simulink model "dcmotor"  (R2021a)
settings: Solver=VariableStepAuto  StartTime=0.0  StopTime=10.0  RelTol=1e-3
undefined symbols (not defined in the file): Ion, Lithium
libraries: spsSeriesRLCBranchLib x5, spsDCMachineLib x1, spsPWMGeneratorDCDCLib x1, spsPVArrayLib x1, spsBatteryLib x1, spsCurrentMeasurementLib x1, spsDiodeLib x1, spsMosfetLib x1, spsVoltageMeasurementLib x1, spspowerguiLib x1
settings Model: Creator=Gue$t  LastModifiedBy=Gue$t

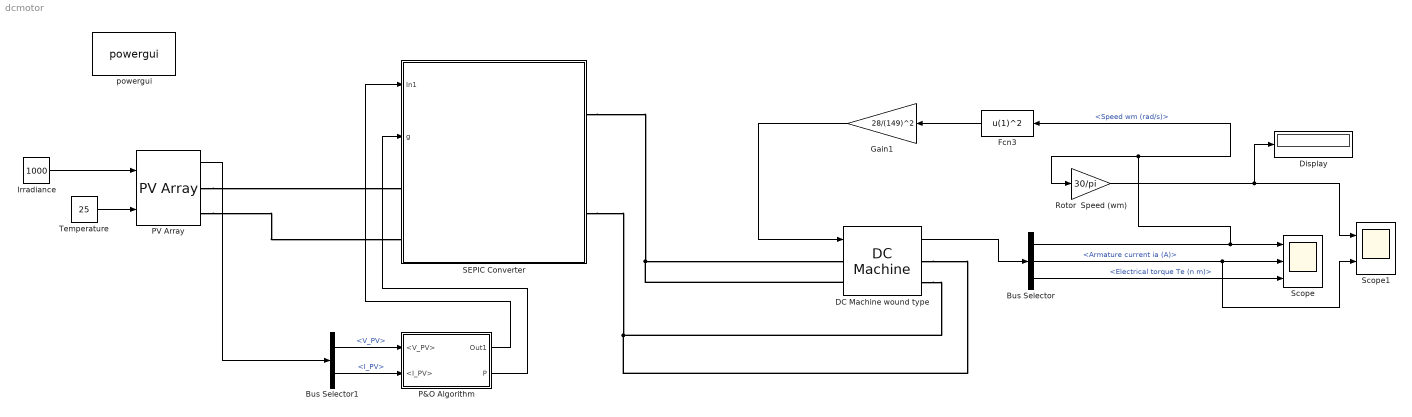
== system dcmotor ==
  Bus Selector : BusSelector  OutputSignals=Speed wm (rad/s),Armature current ia (A),Electrical torque Te (n m)
  Bus Selector1 : BusSelector  OutputSignals=V_PV,I_PV
  DC Machine wound type : spsDCMachineLib/DC Machine  PresetModel=01: 5HP 240V 1750RPM Field:300V  MechanicalLoad=Torque TL  FieldType=Wound  ShowDetailedParameters=on  MeasurementBus=off  RLa=[2.581 0.028]  RLf=[281.2 156]  Laf=0.9483  MachineConstant=Torque constant (N.m/A)  Ke=1.8  Kt=1.8  J=0.02215  Bm=0.002953  Tf=0.5161  w0=1  Ifinit=0  TsPowergui=0  TsBlock=-1
  Display : Display
  Fcn3 : Fcn  Expr=u(1)^2
  Gain1 : Gain  Gain=28/(149)^2
  Irradiance : Constant  Value=1000
  P&O Algorithm : Subsystem
  PV Array : spsPVArrayLib/PV Array  Npar=2  Nser=3  PlotType=array @ 1000 W/m2 & specified temperatures  S_vec="[ 1000  500  100 ]"  Temp_C_vec="[ 45 25  ]"  ModuleName=User-defined  PlotWhenSelected=off  Pm=224.757  Ncell=60  Voc=41.79  Isc=7.13  Vm=33.9  Im=6.63  beta_Voc_pc=-0.36099  alpha_Isc_pc=0.102  beta_Voc=-0.15086  alpha_Isc=0.0072726  IL=7.142  I0=2.6501e-10  nI=1.1299  Rsh=247.0314  Rs=0.41409  RobustModel=off  RobustCellTemperature=313.3991  BAL=on  Tc=1e-6  Tfilter=5e-5
  Rotor  Speed (wm) : Gain  Gain=30/pi
  SEPIC Converter : Subsystem
  Scope : Scope  NumInputPorts=3
  Scope1 : Scope  NumInputPorts=2
  Temperature : Constant  Value=25
  powergui : spspowerguiLib/powergui  Priority=1  SimulationMode=Discrete  SampleTime=1e-6  frequency=60  Iterations=50  frequencyindice=0  Pbase=100e6  ErrMax=1e-4  UnitsV=kV  UnitsW=MW  buscounter=0  FunctionMessages=off  echomessages=off  EnableUseOfTLC=off  CurrentSourceSwitches=off  DisableSnubberDevices=off  DisableRonSwitches=off  DisableVfSwitches=off  DisplayEquations=off  AutomaticDiscreteSolvers=off  SolverType=Tustin/Backward Euler (TBE)  Interpol=off  ExternalGateDelay=off  methode=off  Ts=100  x0status=blocks  SPID=on  SwTol=0  HookPort=off  NonlinearTolerance=0  nMaxIteration=15  ContinueOnMaxIteration=off  RestoreLinks=warning  ResistiveCurrentMeasurement=off  Frange=[0:2:500]  Ylog=off  Xlog=on  ShowGrid=off  save=off  variable=ZData  structure=0  ZoomFFT=off  StartTime=0.0  cycles=1  DisplayStyle=1  fundamental=60  FreqAxis=off  MaxFrequency=1000  frequencyindicesteady=1  RmsSteady=1  display=off
  wires:
  Bus Selector1/2 -> P&O Algorithm/2(<I_PV>)  "<I_PV>"
  PV Array/1 -> Bus Selector1/1
  Irradiance/1 -> PV Array/1
  Bus Selector1/1 -> P&O Algorithm/1(<V_PV>)  "<V_PV>"
  P&O Algorithm/2(P) -> SEPIC Converter/2(g)
  P&O Algorithm/1(Out1) -> SEPIC Converter/1(In1)
  Temperature/1 -> PV Array/2
  Bus Selector/3 -> Scope/3  "<Electrical torque Te (n m)>"
  Fcn3/1 -> Gain1/1
  Bus Selector/1 -> Fcn3/1, Rotor  Speed (wm)/1, Scope/1  "<Speed wm (rad/s)>"
  Rotor  Speed (wm)/1 -> Scope1/1, Display/1
  Bus Selector/2 -> Scope1/2, Scope/2  "<Armature current ia (A)>"
  DC Machine wound type/1 -> Bus Selector/1
  Gain1/1 -> DC Machine wound type/1
  connections:
  PV Array/RConn1 -- SEPIC Converter/LConn1
  PV Array/RConn2 -- SEPIC Converter/LConn2
  SEPIC Converter/RConn2 -- DC Machine wound type/RConn1 -- DC Machine wound type/RConn2
  SEPIC Converter/RConn1 -- DC Machine wound type/LConn2 -- DC Machine wound type/LConn1

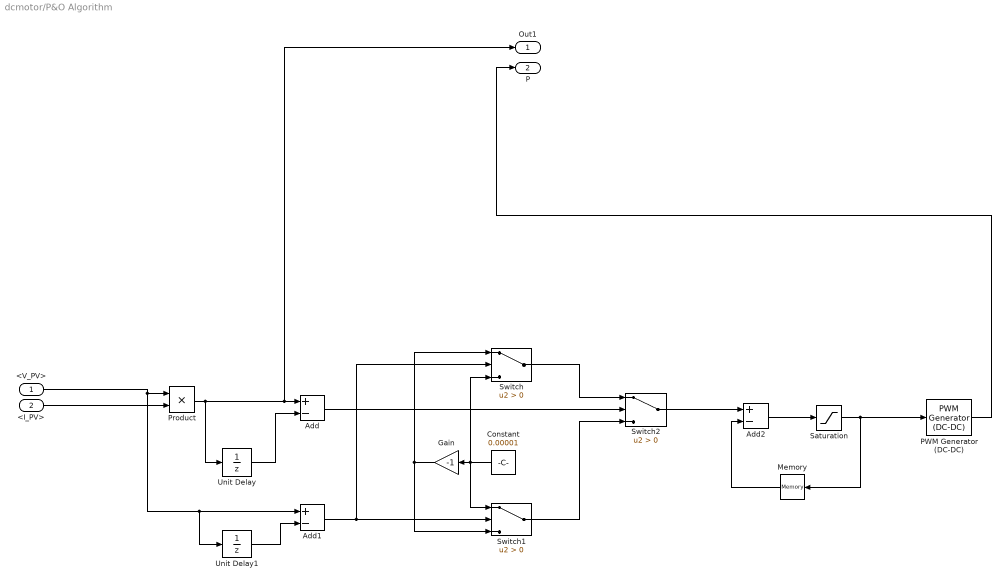
== system dcmotor/P&O Algorithm ==
  <V_PV> : Inport
  <I_PV> : Inport  Port=2
  Add : Sum  Inputs=+-
  Add1 : Sum  Inputs=+-
  Add2 : Sum  Inputs=+-
  Constant : Constant  Value=0.00001
  Gain : Gain  Gain=-1
  Memory : Memory
  PWM Generator (DC-DC) : spsPWMGeneratorDCDCLib/PWM Generator (DC-DC)  Fsw=50  Ts=0
      link override Sawtooth Generator/Model/Hit  Crossing: HitCrossingOffset=0.001
  Product : Product
  Saturation : Saturate
  Switch : Switch  Criteria=u2 > Threshold
  Switch1 : Switch  Criteria=u2 > Threshold
  Switch2 : Switch  Criteria=u2 > Threshold
  Unit Delay : UnitDelay  SampleTime=-1  HasFrameUpgradeWarning=on
  Unit Delay1 : UnitDelay  SampleTime=-1  HasFrameUpgradeWarning=on
  Out1 : Outport
  P : Outport  Port=2
  wires:
  Add1/1 -> Switch/2, Switch1/2
  Constant/1 -> Switch1/1, Switch/3, Gain/1
  Product/1 -> Out1/1, Add/1, Unit Delay/1
  Gain/1 -> Switch1/3, Switch/1
  Switch/1 -> Switch2/1
  PWM Generator (DC-DC)/1 -> P/1
  Switch2/1 -> Add2/1
  Add/1 -> Switch2/2
  Switch1/1 -> Switch2/3
  Saturation/1 -> Memory/1, PWM Generator (DC-DC)/1
  <V_PV>/1 -> Add1/1, Unit Delay1/1, Product/1
  Unit Delay1/1 -> Add1/2
  Add2/1 -> Saturation/1
  Unit Delay/1 -> Add/2
  Memory/1 -> Add2/2
  <I_PV>/1 -> Product/2

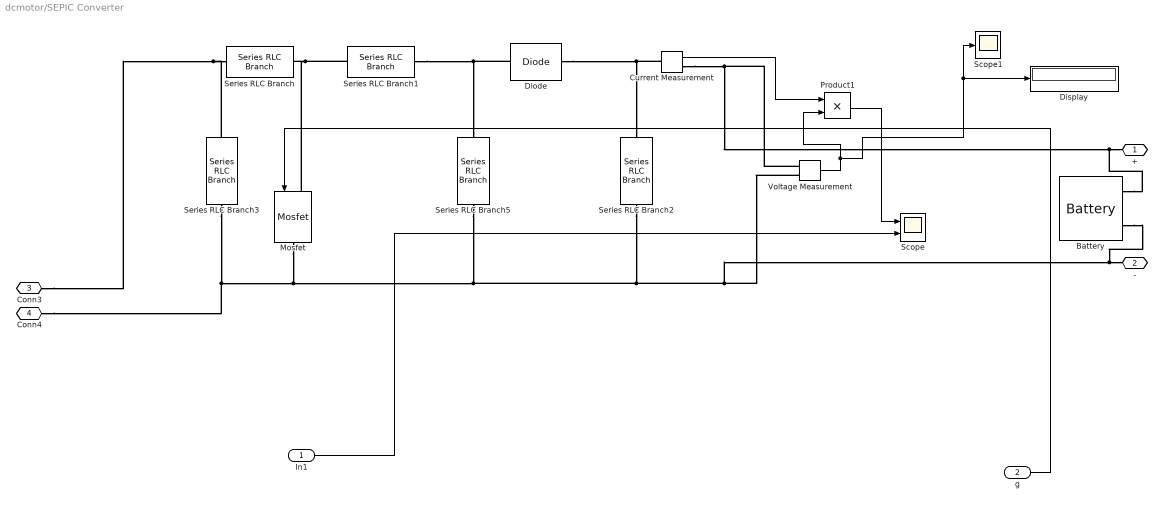
== system dcmotor/SEPIC Converter ==
  In1 : Inport
  g : Inport  Port=2
  Battery : spsBatteryLib/Battery  BatType=Lithium-Ion  ShowTempParam=off  ThermalPreset=no  ShowAgeParam=off  NomV=350  NomQ=5.4  SOC=100  Batt_Tr=30  PresetModel=on  MaxQ=5.4  MinV=262.5  FullV=407.3955  Dis_rate=2.3478  R=0.64815  Normal_OP=4.8835  expZone="[378.135     0.2653043]"  current=[6.5 13 32.5]  Units=Time  Tci=20  NomT=20  T2=-30  MaxQ2=4.8  FullV2=7.1  Normal_OP2=5.655  expZone2="[6.58           1]"  Rca=0.6  ti=2000  Dp=0  Neq0=0  Tsim=1e6  Ta1=25  Qeol=5.4*0.9  Reol=0.013333*1.2  Char_age=[2.3478, 3]  Dis_age=[2.3478, 10]  N1=1500  N2=10500  N3=1000  N4=1400  Ta2=45  N5=950
  Current Measurement : spsCurrentMeasurementLib/Current Measurement  PhasorSimulation=off  OutputType=Complex  PSBequivalent=0
  Diode : spsDiodeLib/Diode  Ron=0.001  Lon=0  Vf=0.8  IC=0  UseSnubber=0  Rs=500  Cs=250e-9  Measurements=off
  Display : Display
  Mosfet : spsMosfetLib/Mosfet  Ron=0.1  Lon=0  Rd=0.01  Vfd=0  IC=0  Rs=1e5  Cs=inf  Measurements=off
  Product1 : Product
  Scope : Scope  NumInputPorts=2
  Scope1 : Scope
  Series RLC Branch : spsSeriesRLCBranchLib/Series RLC Branch  LConnTagsString=__new0  RConnTagsString=__new0  BranchType=L  Resistance=1  Inductance=2.12e-3  SetiL0=off  InitialCurrent=0  Capacitance=1e-6  Setx0=off  InitialVoltage=0  Measurements=None
  Series RLC Branch1 : spsSeriesRLCBranchLib/Series RLC Branch  LConnTagsString=__new0  RConnTagsString=__new0  BranchType=C  Resistance=1  Inductance=1e-3  SetiL0=off  InitialCurrent=0  Capacitance=1100e-6  Setx0=off  InitialVoltage=0  Measurements=None
  Series RLC Branch2 : spsSeriesRLCBranchLib/Series RLC Branch  LConnTagsString=__new0  RConnTagsString=__new0  BranchType=C  Resistance=1  Inductance=1e-3  SetiL0=off  InitialCurrent=0  Capacitance=1100e-6  Setx0=off  InitialVoltage=0  Measurements=None
  Series RLC Branch3 : spsSeriesRLCBranchLib/Series RLC Branch  LConnTagsString=__new0  RConnTagsString=__new0  BranchType=C  Resistance=1  Inductance=1e-3  SetiL0=off  InitialCurrent=0  Capacitance=1100e-6  Setx0=off  InitialVoltage=0  Measurements=None
  Series RLC Branch5 : spsSeriesRLCBranchLib/Series RLC Branch  LConnTagsString=__new0  RConnTagsString=__new0  BranchType=L  Resistance=1  Inductance=2.12e-3  SetiL0=off  InitialCurrent=0  Capacitance=1e-6  Setx0=off  InitialVoltage=0  Measurements=None
  Voltage Measurement : spsVoltageMeasurementLib/Voltage Measurement  PhasorSimulation=off  OutputType=Complex  PSBequivalent=0
  + : PMIOPort  Side=Right
  - : PMIOPort  Port=2  Side=Right
  Conn3 : PMIOPort  Port=3  Side=Left
  Conn4 : PMIOPort  Port=4  Side=Left
  wires:
  Voltage Measurement/1 -> Product1/2, Scope1/1, Display/1
  Product1/1 -> Scope/1
  g/1 -> Mosfet/1
  Current Measurement/1 -> Product1/1
  In1/1 -> Scope/2
  connections:
  Series RLC Branch1/LConn1 -- Mosfet/LConn1 -- Series RLC Branch/RConn1
  Current Measurement/LConn1 -- Diode/RConn1 -- Series RLC Branch2/LConn1
  Series RLC Branch3/LConn1 -- Series RLC Branch/LConn1 -- Conn3/RConn1
  Series RLC Branch1/RConn1 -- Diode/LConn1 -- Series RLC Branch5/LConn1
  Current Measurement/RConn1 -- Voltage Measurement/LConn1 -- Battery/LConn1 -- +/RConn1
  Mosfet/RConn1 -- Series RLC Branch5/RConn1 -- Voltage Measurement/LConn2 -- Battery/LConn2 -- -/RConn1 -- Series RLC Branch2/RConn1 -- Series RLC Branch3/RConn1 -- Conn4/RConn1
